simulink model "s0232"  (Simulink 6.0)
settings: Solver=ode45  SolverMode=SingleTasking  StartTime=0.0  StopTime=999999  MaxStep=10  RelTol=1e-3  AbsTol=1e-6
values from neighbouring files (symbols this model uses):
  nen1 = Gs1.den{1}    [m0232.m]
  nen2 = Gs2.den{1}    [m0232.m]
  zae1 = Gs1.num{1}    [m0232.m]
  zae2 = Gs2.num{1}    [m0232.m]
settings Model: LastModifiedBy=Froriep
settings DataIOCC: LimitDataPoints=off  SaveOutput=off  SaveTime=off
settings OptimizationCC: BooleanDataType=off
settings DebuggingCC: SolverPrmCheckMsg=none
settings HardwareCC: TargetUnknown=on
settings STFCustomTargetCC: TargetFcnLib=ansi_tfl_tmw.mat  GenFloatMathFcnCalls=ANSI_C  ModelReferenceCompliant=off  SystemTargetFile=grt.tlc

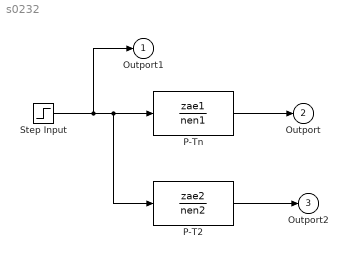
== system s0232 ==
  P-T2 : TransferFcn  Numerator=zae2  Denominator=nen2
  P-Tn : TransferFcn  Numerator=zae1  Denominator=nen1
  Step Input : Step  Time=.001  SampleTime=0
  Outport1 : Outport
  Outport : Outport  Port=2
  Outport2 : Outport  Port=3
  wires:
  P-T2/1 -> Outport2/1
  Step Input/1 -> P-T2/1, P-Tn/1, Outport1/1
  P-Tn/1 -> Outport/1
